simulink model "Lab1A_C2"  (R2019b)
settings: Solver=VariableStepAuto  StartTime=0.0  StopTime=10.0  RelTol=1e-3
settings Model: Creator=sinow  LastModifiedBy=sinow

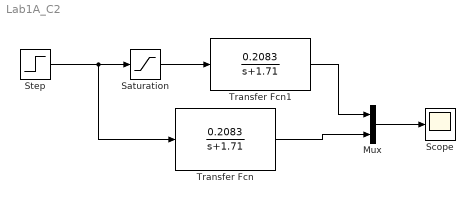
== system Lab1A_C2 ==
  Mux : Mux  Inputs=2
  Saturation : Saturate  UpperLimit=5  LowerLimit=-5
  Scope : Scope
  Step : Step  Time=0  After=10  SampleTime=0
  Transfer Fcn : TransferFcn  Numerator=0.2083  Denominator=[1 1.71]
  Transfer Fcn1 : TransferFcn  Numerator=0.2083  Denominator=[1 1.71]
  wires:
  Step/1 -> Transfer Fcn/1, Saturation/1
  Saturation/1 -> Transfer Fcn1/1
  Transfer Fcn/1 -> Mux/2
  Transfer Fcn1/1 -> Mux/1
  Mux/1 -> Scope/1
